simulink model "Traffic_Light"  (R2021a)
settings: Solver=FixedStepDiscrete  StartTime=0.0  StopTime=20  RelTol=1e-3  EnableMultiTasking=on
settings Model: Creator=omar  LastModifiedBy=omar
settings DataIOCC: ReturnWorkspaceOutputs=off
settings OptimizationCC: DefaultParameterBehavior=Inlined  InlineInvariantSignals=on  EnableMemcpy=off  LifeSpan=1  EfficientTunableParamExpr=on
settings DebuggingCC: UnderspecifiedInitializationDetection=Classic  MergeDetectMultiDrivingBlocksExec=none  SFMachineParentedDataDiag=warning  ArithmeticOperatorsInVariantConditions=warning
settings ModelReferenceCC: PropagateSignalLabelsOutOfModel=off
settings SFSimCC: MATLABDynamicMemAlloc=off  CustomCodeUndefinedFunction=UseInterfaceOnly
settings RTWCC: SystemTargetFile=ert.tlc  GenCodeOnly=on  TemplateMakefile=ert_default_tmf  GenerateReport=on  IncludeHyperlinkInReport=on  LaunchReport=on  GenerateTraceInfo=on  GenerateTraceReport=on  GenerateTraceReportSl=on  GenerateTraceReportSf=on  GenerateTraceReportEml=on
settings CodeAppCC: ForceParamTrailComments=on  IgnoreCustomStorageClasses=off  OperatorAnnotations=on  SimulinkDataObjDesc=on  SFDataObjDesc=on  MATLABFcnDesc=on  InsertBlockDesc=on  StateflowObjectComments=on  MATLABSourceComments=on
settings ERTTargetCC: MultiwordLength=2048  GenerateSampleERTMain=on  InlinedParameterPlacement=NonHierarchical  ERTCustomFileTemplate=example_file_process.tlc

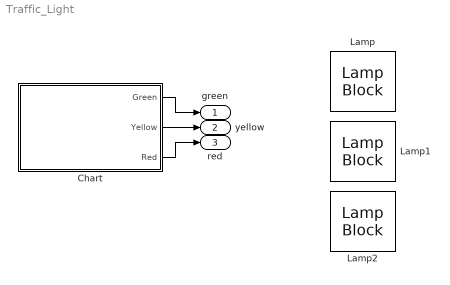
== system Traffic_Light ==
  Chart : Stateflow chart  TreatAsAtomicUnit=on
  Lamp : LampBlock  LabelPosition=Hide
  Lamp1 : LampBlock  LabelPosition=Hide
  Lamp2 : LampBlock  LabelPosition=Hide
  green : Outport  SignalName=Green
  yellow : Outport  Port=2  SignalName=Yellow
  red : Outport  Port=3  SignalName=Red
  wires:
  Chart/1(Green) -> green/1
  Chart/2(Yellow) -> yellow/1
  Chart/3(Red) -> red/1

== stateflow chart Traffic_Light/Chart ==
  state Stop
    entry:
    Red = 1;
    Yellow = 0;
    Green = 0;
  state PrepareToStop
    entry:
    Red = 0;
    Yellow = 1;
    Green = 0;
  state Go
    entry:
    Red = 0;
    Yellow = 0;
    Green = 1;
  (default) -> Stop
  Go -> Stop : after(3,sec)
  Stop -> PrepareToStop : after(3,sec)
  PrepareToStop -> Go : after(3,sec)
  data: Green output =0; Yellow output =0; Red output =0
